simulink model "pathFollowing"  (R2023a)
settings: Solver=FixedStepDiscrete  StartTime=0.0  StopTime=Inf  FixedStep=0.1  RelTol=1e-3  EnableMultiTasking=on
StopFcn:
  | 
  |  % Do not delete, this is an auto-generated function to log ROS message.
  |  ros.slros.internal.ROSUtil.logROSMessageToBagFile(bdroot);
model workspace (MAT data in the model file):
  ROSLoggingInfo_.GenBagFile = 1
  ROSLoggingInfo_.BagFileName = 'pathFollowing'
  ROSLoggingInfo_.CompressionFormat = 'uncompressed'
  ROSLoggingInfo_.ChunkSize = 786432
  ROSLoggingInfo_.LogOption = 'Default'
  ROSLoggingInfo_.FilePrefix = ''
  ROSLoggingReload_{1,1} = 'pathFollowing/Altitude controller/Subscribe1'
  ROSLoggingReload_{2,1} = 'pathFollowing/Cameras/Subscribe2'
  ROSLoggingReload_{3,1} = 'pathFollowing/Cameras/Subscribe3'
  ROSLoggingReload_{4,1} = 'pathFollowing/Output/Blank Message'
  ROSLoggingReload_{5,1} = 'pathFollowing/Robot position/Subscribe1'
  ROSLoggingReload_{6,1} = 'pathFollowing/Altitude controller/Extract Position.Z/Msg'
  ROSLoggingReload_{7,1} = 'pathFollowing/Output/Bus
    | Assignment'
  ROSLoggingReload_{8,1} = 'pathFollowing/Robot position/Subsystem/In1'
  ROSLoggingReload_{1,2} = 0
  ROSLoggingReload_{2,2} = 0
  ROSLoggingReload_{3,2} = 0
  ROSLoggingReload_{4,2} = 0
  ROSLoggingReload_{5,2} = 1
  ROSLoggingReload_{6,2} = 0
  ROSLoggingReload_{7,2} = 0
  ROSLoggingReload_{8,2} = 0
  ROSLoggingReload_{1,3} = 'quadrotor_1_ground_truth_state_altitude_controller_subscribe1'
  ROSLoggingReload_{2,3} = 'quadrotor_1_front_image_raw_cameras_subscribe2'
  ROSLoggingReload_{3,3} = 'quadrotor_1_bottom_image_raw_cameras_subscribe3'
  ROSLoggingReload_{4,3} = 'output_blank_message'
  ROSLoggingReload_{5,3} = 'quadrotor_1_ground_truth_state_robot_position_subscribe1'
  ROSLoggingReload_{6,3} = []
  ROSLoggingReload_{7,3} = 'quadrotor_1/cmd_vel_output_bus_assignment'
  ROSLoggingReload_{8,3} = 'robot_position_subsystem_in1'
  ROSLoggingTable_ = {1, 'Robot position/Subscribe1:2', 'quadrotor_1_ground_truth_state_robot_position_subscribe1', 'nav_msgs/Odometry'}
  SL_ROS_VariableLengthArrays_MaxSizes.CommonInfo.ArrayTruncateAction = 'EmitWarning'
  SL_ROS_VariableLengthArrays_MaxSizes.MsgTypeMap = containers.Map
  SL_ROS_VariableLengthArrays_MaxSizes.MsgTypeMap.serialization.keys = {'sensor_msgs/Image', 'sensor_msgs/LaserScan'}
  SL_ROS_VariableLengthArrays_MaxSizes.MsgTypeMap.serialization.values{1}(1).PropertyName = 'Data'
  SL_ROS_VariableLengthArrays_MaxSizes.MsgTypeMap.serialization.values{1}(1).DataType = 'uint8'
  SL_ROS_VariableLengthArrays_MaxSizes.MsgTypeMap.serialization.values{1}(1).MaxLength = 691200
  SL_ROS_VariableLengthArrays_MaxSizes.MsgTypeMap.serialization.values{1}(2).PropertyName = 'Encoding'
  SL_ROS_VariableLengthArrays_MaxSizes.MsgTypeMap.serialization.values{1}(2).DataType = 'uint8'
  SL_ROS_VariableLengthArrays_MaxSizes.MsgTypeMap.serialization.values{1}(2).MaxLength = 128
  SL_ROS_VariableLengthArrays_MaxSizes.MsgTypeMap.serialization.values{2}(1).PropertyName = 'Intensities'
  SL_ROS_VariableLengthArrays_MaxSizes.MsgTypeMap.serialization.values{2}(1).DataType = 'single'
  SL_ROS_VariableLengthArrays_MaxSizes.MsgTypeMap.serialization.values{2}(1).MaxLength = 1081
  SL_ROS_VariableLengthArrays_MaxSizes.MsgTypeMap.serialization.values{2}(2).PropertyName = 'Ranges'
  SL_ROS_VariableLengthArrays_MaxSizes.MsgTypeMap.serialization.values{2}(2).DataType = 'single'
  SL_ROS_VariableLengthArrays_MaxSizes.MsgTypeMap.serialization.values{2}(2).MaxLength = 1081
  SL_ROS_VariableLengthArrays_MaxSizes.MsgTypeMap.serialization.uniformity = 0
  SL_ROS_VariableLengthArrays_MaxSizes.MsgTypeMap.serialization.keyType = 'char'
  SL_ROS_VariableLengthArrays_MaxSizes.MsgTypeMap.serialization.valueType = 'any'
undefined symbols (not defined in the file): Angular, gray, Linear
libraries: robotlib x8, slpidlib x1, robotalgslib x1, aerolibanimutils x1
settings Model: Creator=The MathWorks, Inc.  LastModifiedBy=root
settings SolverCC: AlgebraicLoopSolver=TrustRegion
settings DataIOCC: LimitDataPoints=on  SaveFormat=Array  ReturnWorkspaceOutputs=off
settings OptimizationCC: LifeSpan=Inf  MaxStackSize=64
settings DebuggingCC: SolverPrmCheckMsg=warning  UnconnectedInputMsg=warning  UnconnectedOutputMsg=warning  UnconnectedLineMsg=warning  SFUnexpectedBacktrackingDiag=warning  SFNoUnconditionalDefaultTransitionDiag=warning  SFExecutionAtInitializationDiag=none  ArithmeticOperatorsInVariantConditions=warning
settings HardwareCC: ProdBitPerPointer=32  ProdBitPerSizeT=32  ProdBitPerPtrDiffT=32  ProdLargestAtomicFloat=None  ProdIntDivRoundTo=Undefined  ProdEndianess=Unspecified  ProdWordSize=32  ProdHWDeviceType=Generic->Unspecified (assume 32-bit Generic)  UseEmbeddedCoderFeatures=off
settings ModelReferenceCC: EnableRefExpFcnMdlSchedulingChecks=on  PropagateSignalLabelsOutOfModel=off
settings SFSimCC: SimUseLocalCustomCode=off  CustomCodeUndefinedFunction=UseInterfaceOnly  SimTargetLang=C++
settings RTWCC: Description=Embedded Coder  SystemTargetFile=ert.tlc  HardwareBoard=Robot Operating System (ROS)  TLCOptions=-aInlineSetEventsForThisBaseRateFcn=TLC_FALSE -aSuppressMultiTaskScheduler=TLC_FALSE -aRateBasedStepFcn=0  TemplateMakefile=ert_default_tmf  RTWUseLocalCustomCode=off  Toolchain=Catkin  TargetLang=C++
settings CodeAppCC: StateflowObjectComments=on
settings ERTTargetCC: MultiwordLength=2048  ERTCustomFileBanners=off  SupportContinuousTime=on  SupportNonInlinedSFcns=on  RemoveResetFunc=off  SupportVariableSizeSignals=on  ModelStepFunctionPrototypeControlCompliant=off  ConvertIfToSwitch=off  SuppressUnreachableDefaultCases=off
settings ConfigComp: CovMetricSettings=dw  CovSaveCumulativeToWorkspaceVar=on  CovSaveSingleToWorkspaceVar=on  CovExternalEMLEnable=off  CovSFcnEnable=off

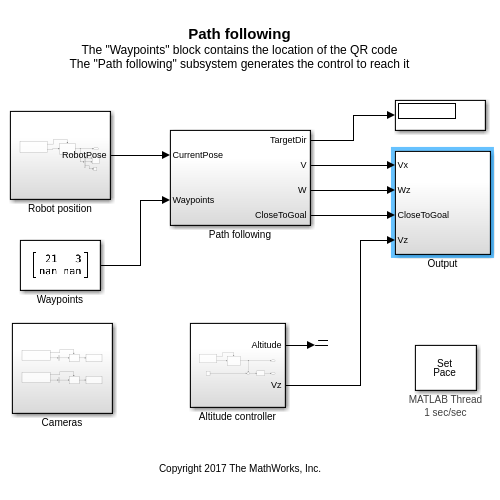
[thumbnail: Simulink's stored preview of the top-level diagram]
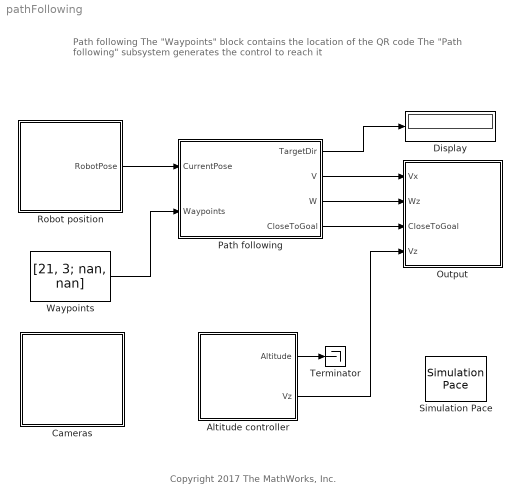
== system pathFollowing ==
  note: Path following
      | The "Waypoints" block contains the location of the QR code
      | The "Path following" subsystem generates the control to reach it
  note: Copyright 2017 The MathWorks, Inc.
  Altitude controller : Subsystem
  Cameras : Subsystem
  Display : Display
  Output : Subsystem
  Path following : Subsystem
  Robot position : Subsystem
  Simulation Pace : aerolibanimutils/Simulation Pace  SimulationPace=1  SleepMode=MATLAB Thread  OutputPaceError=off  SampleTime=-1
  Terminator : Terminator
  Waypoints : Constant  Value=[21, 3; nan, nan]  OutDataTypeStr=double
  wires:
  Waypoints/1 -> Path following/2(Waypoints)
  Path following/2(V) -> Output/1(Vx)
  Path following/4(CloseToGoal) -> Output/3(CloseToGoal)
  Path following/3(W) -> Output/2(Wz)
  Path following/1(TargetDir) -> Display/1
  Robot position/1(RobotPose) -> Path following/1(CurrentPose)
  Altitude controller/2(Vz) -> Output/4(Vz)
  Altitude controller/1(Altitude) -> Terminator/1

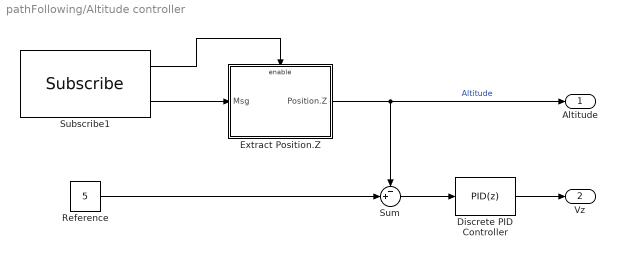
== system pathFollowing/Altitude controller ==
  Discrete PID Controller : slpidlib/PID Controller  Controller=PID  Form=Parallel  TimeDomain=Discrete-time  UseExternalTs=off  SampleTime=-1  IntegratorMethod=Forward Euler  FilterMethod=Forward Euler  ControllerParametersSource=internal  P=1  I=0  UseKiTs=off  D=0  N=100  UseFilter=on  TunerSelectOption=Transfer Function Based (PID Tuner App)  InitialConditionSource=internal  InitialConditionForIntegrator=0  InitialConditionForFilter=0  DifferentiatorICPrevScaledInput=0  ExternalReset=none  TrackingMode=off  Kt=1  LimitOutput=on  SatLimitsSource=internal  UpperSaturationLimit=1  LowerSaturationLimit=-1  LinearizeAsGain=off  AntiWindupMode=none  Kb=1  LimitIntegrator=off  UpperIntegratorSaturationLimit=inf  LowerIntegratorSaturationLimit=-inf  POutMin=[]  POutMax=[]  IOutMin=[]  IOutMax=[]  DOutMin=[]  DOutMax=[]  NOutMin=[]  NOutMax=[]  SumOutMin=[]  SumOutMax=[]  SaturationOutMin=[]  SaturationOutMax=[]  PParamMin=[]  PParamMax=[]  IParamMin=[]  IParamMax=[]  DParamMin=[]  DParamMax=[]  NParamMin=[]  NParamMax=[]  KbParamMin=[]  KbParamMax=[]  KtParamMin=[]  KtParamMax=[]  KbOutMin=[]  KbOutMax=[]  KtOutMin=[]  KtOutMax=[]  IntegratorOutMin=[]  IntegratorOutMax=[]  FilterOutMin=[]  FilterOutMax=[]  SumI1OutMin=[]  SumI1OutMax=[]  SumI2OutMin=[]  SumI2OutMax=[]  SumI3OutMin=[]  SumI3OutMax=[]  SumI4OutMin=[]  SumI4OutMax=[]  SumDOutMin=[]  SumDOutMax=[]  DifferentiatorOutMin=[]  DifferentiatorOutMax=[]  FilterDiffOutCoefMin=[]  FilterDiffOutCoefMax=[]  ReciprocalOutMin=[]  ReciprocalOutMax=[]  SumDenOutMin=[]  SumDenOutMax=[]  SumNumOutMin=[]  SumNumOutMax=[]  DivideOutMin=[]  DivideOutMax=[]  UdiffTsProdOutMin=[]  UdiffTsProdOutMax=[]  NTsProdOutMin=[]  NTsProdOutMax=[]  UintegralTsProdOutMin=[]  UintegralTsProdOutMax=[]  UngainTsProdOutMin=[]  UngainTsProdOutMax=[]  ClampingZeroOutDataTypeStr=Inherit: Inherit via back propagation  ClampingZeroOutMin=[]  ClampingZeroOutMax=[]  FilterDenConstantOutDataTypeStr=Inherit: Inherit via back propagation  FilterDenConstantOutMin=[]  FilterDenConstantOutMax=[]  PCopyOutDataTypeStr=Inherit: Inherit via back propagation  PCopyOutMin=[]  PCopyOutMax=[]  NCopyOutDataTypeStr=Inherit: Inherit via back propagation  NCopyOutMin=[]  NCopyOutMax=[]  IntegratorContinuousStateAttributes=''  IntegratorStateMustResolveToSignalObject=off  IntegratorRTWStateStorageClass=Auto  FilterContinuousStateAttributes=''  FilterStateMustResolveToSignalObject=off  FilterRTWStateStorageClass=Auto  ParallelPVariant=InternalParameters  IdealPVariant=Disabled  IVariant=InternalParameters  DVariant=InternalParameters  IntegratorVariant=Discrete  SatVariant=Enabled  AWVariant=Passthrough  PCopyVariant=Disabled  TRVariant=Disabled  FdbkBlocksVariant=Forward  IdealPFdbkVariant=Disabled  SatFdbkVariant=Disabled  DerivativeFilterVariant=ForwardEulerFilter  NVariant=InternalParameters  NCopyVariant=Disabled  FilterICVariant=InternalICsFilter  IntegratorICVariant=InternalICs  ExternalResetVariant=Disabled  TRSumVariant=Passthrough  SumFdbkVariant=Disabled  SumVariant=Sum_PID  TsampFilterVariant=InternalTs  TsampNgainVariant=Passthrough  TsampIntegralVariant=Disabled_SignalSpec  ExternalSaturationOutDataTypeStr=Inherit: Same as second input
  Extract Position.Z : Subsystem
  Reference : Constant  Value=5
  Subscribe1 : robotlib/Subscribe  topicSource=Select from ROS network  topic=/quadrotor_1/ground_truth/state  messageType=nav_msgs/Odometry  SampleTime=-1  legacyBusStruct=off  messageQueueLength=51
  Sum : Sum  Inputs=-+|
  Altitude : Outport
  Vz : Outport  Port=2
  wires:
  Subscribe1/1 -> Extract Position.Z/Enable
  Subscribe1/2 -> Extract Position.Z/1(Msg)
  Sum/1 -> Discrete PID Controller/1
  Reference/1 -> Sum/2
  Extract Position.Z/1(Position.Z) -> Altitude/1, Sum/1  "Altitude"
  Discrete PID Controller/1 -> Vz/1

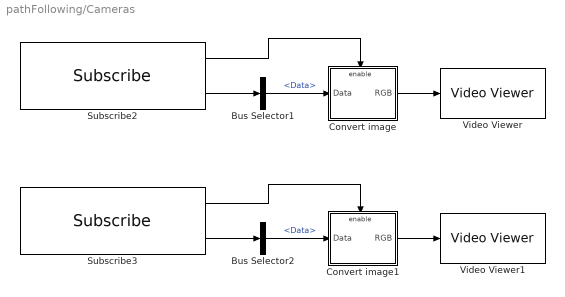
== system pathFollowing/Cameras ==
  Bus Selector1 : BusSelector  DialogController=Simulink.DDGSource_BusSelector  OutputSignals=Data
  Bus Selector2 : BusSelector  DialogController=Simulink.DDGSource_BusSelector  OutputSignals=Data
  Convert image : Subsystem
  Convert image1 : Subsystem
  Subscribe2 : robotlib/Subscribe  topicSource=Select from ROS network  topic=/quadrotor_1/front/image_raw  messageType=sensor_msgs/Image  SampleTime=-1  legacyBusStruct=off  messageQueueLength=51
  Subscribe3 : robotlib/Subscribe  topicSource=Select from ROS network  topic=/quadrotor_1/bottom/image_raw  messageType=sensor_msgs/Image  SampleTime=-1  legacyBusStruct=off  messageQueueLength=51
  Video Viewer : VideoViewer  colormapValue=gray(256)  FigPos=[252 563 599 376]
  Video Viewer1 : VideoViewer  colormapValue=gray(256)  FigPos=[964 607 629 376]
  wires:
  Subscribe2/1 -> Convert image/Enable
  Convert image1/1(RGB) -> Video Viewer1/1
  Subscribe3/2 -> Bus Selector2/1
  Subscribe2/2 -> Bus Selector1/1
  Bus Selector1/1 -> Convert image/1(Data)  "<Data>"
  Bus Selector2/1 -> Convert image1/1(Data)  "<Data>"
  Subscribe3/1 -> Convert image1/Enable
  Convert image/1(RGB) -> Video Viewer/1

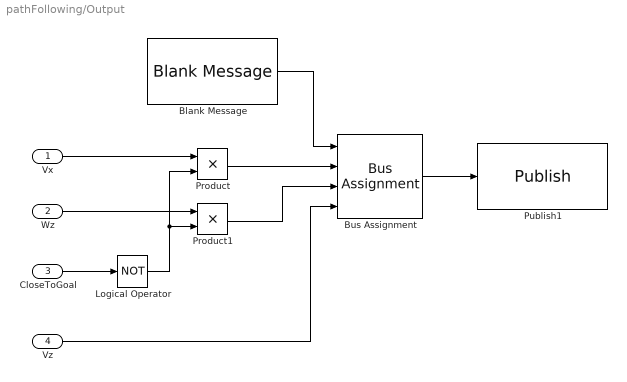
== system pathFollowing/Output ==
  Vx : Inport
  Wz : Inport  Port=2
  CloseToGoal : Inport  Port=3
  Vz : Inport  Port=4
  Blank Message : robotlib/Blank Message  messageClass=Message  entityType=geometry_msgs/Twist  messageType=geometry_msgs/Twist  SampleTime=0  legacyBusStruct=off
  Bus Assignment : BusAssignment  DialogController=Simulink.DDGSource_BusAssignment  AssignedSignals=Linear.X,Angular.Z,Linear.Z
  Logical Operator : Logic  Operator=NOT  AllPortsSameDT=off  OutDataTypeStr=boolean
  Product : Product
  Product1 : Product
  Publish1 : robotlib/Publish  topicSource=Select from ROS network  topic=/quadrotor_1/cmd_vel  messageType=geometry_msgs/Twist  legacyBusStruct=off  messageQueueLength=105
  wires:
  Bus Assignment/1 -> Publish1/1
  Blank Message/1 -> Bus Assignment/1
  Logical Operator/1 -> Product1/2, Product/2
  Product1/1 -> Bus Assignment/3
  CloseToGoal/1 -> Logical Operator/1
  Product/1 -> Bus Assignment/2
  Vx/1 -> Product/1
  Wz/1 -> Product1/1
  Vz/1 -> Bus Assignment/4

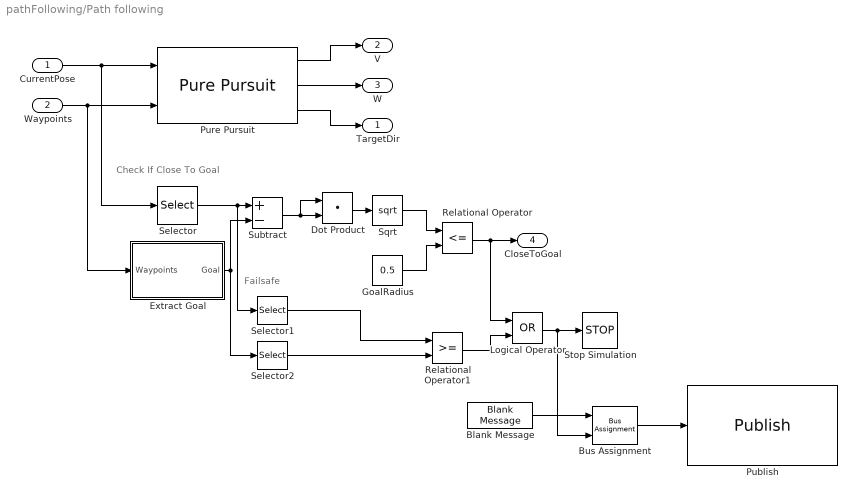
== system pathFollowing/Path following ==
  note: Check If Close To Goal
  note: Failsafe
  CurrentPose : Inport
  Waypoints : Inport  Port=2
  " Extract Goal" : MATLAB Function  TreatAsAtomicUnit=on
  Blank Message : robotlib/Blank Message  messageClass=Message  entityType=std_msgs/Bool  messageType=std_msgs/Bool  SampleTime=inf  legacyBusStruct=off
  Bus Assignment : BusAssignment  AssignedSignals=Data
  Dot Product : DotProduct  OutDataTypeStr=Inherit: Inherit via internal rule
  GoalRadius : Constant  Value=0.5
  Logical Operator : Logic  Operator=OR  AllPortsSameDT=off  OutDataTypeStr=boolean
  Publish : robotlib/Publish  topicSource=Specify your own  topic=/pause_gazebo_topic  messageType=std_msgs/Bool  legacyBusStruct=off  messageQueueLength=1
  Pure Pursuit : robotalgslib/Pure Pursuit  DesiredLinearVelocity=0.3  MaxAngularVelocity=1.0  LookaheadDistance=2.0  TargetDirPort=on  SimulateUsing=Code generation
  Relational Operator : RelationalOperator  Operator=<=  OutDataTypeStr=boolean  RndMeth=Simplest  InputSameDT=off
  Relational Operator1 : RelationalOperator  OutDataTypeStr=boolean  RndMeth=Simplest  InputSameDT=off
  Selector : Selector  InputPortWidth=3  IndexOptions=Index vector (dialog)  Indices=[1 2]  OutputSizes=1
  Selector1 : Selector  InputPortWidth=2  IndexOptions=Index vector (dialog)  Indices=[1]  OutputSizes=1
  Selector2 : Selector  InputPortWidth=2  IndexOptions=Index vector (dialog)  Indices=[1]  OutputSizes=1
  Sqrt : Sqrt
  Stop Simulation : Stop
  Subtract : Sum  Inputs=+-
  TargetDir : Outport
  V : Outport  Port=2
  W : Outport  Port=3
  CloseToGoal : Outport  Port=4
  wires:
  Pure Pursuit/3 -> TargetDir/1
  Pure Pursuit/2 -> W/1
  Pure Pursuit/1 -> V/1
  " Extract Goal"/1(Goal) -> Subtract/2, Selector2/1
  Waypoints/1 -> " Extract Goal"/1(Waypoints), Pure Pursuit/2
  CurrentPose/1 -> Selector/1, Pure Pursuit/1
  GoalRadius/1 -> Relational Operator/2
  Selector/1 -> Selector1/1, Subtract/1
  Dot Product/1 -> Sqrt/1
  Sqrt/1 -> Relational Operator/1
  Subtract/1 -> Dot Product/1, Dot Product/2
  Relational Operator/1 -> Logical Operator/1, CloseToGoal/1
  Logical Operator/1 -> Bus Assignment/2, Stop Simulation/1
  Selector1/1 -> Relational Operator1/1
  Selector2/1 -> Relational Operator1/2
  Relational Operator1/1 -> Logical Operator/2
  Blank Message/1 -> Bus Assignment/1
  Bus Assignment/1 -> Publish/1

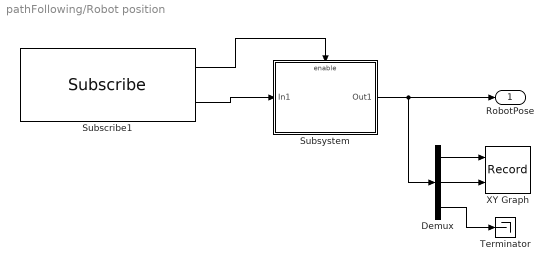
== system pathFollowing/Robot position ==
  Demux : Demux  Outputs=3
  Subscribe1 : robotlib/Subscribe  topicSource=Select from ROS network  topic=/quadrotor_1/ground_truth/state  messageType=nav_msgs/Odometry  SampleTime=-1  legacyBusStruct=off  messageQueueLength=51
  Subsystem : Subsystem
  Terminator : Terminator
  XY Graph : Record  FileSettingsInternal="{\"entries\":[{\"content\":{\"excelSettings\":{\"content\":{},\"type\":\"Streamout.ExcelSettings\"}},\"type\":\"Streamout.FileSettingStorage\",\"uuid\":\"\"}],\"packageUris\":[\"http:\\/\\/schema.mathworks.com\\/mf0\\/streamout_blocks\\/R2020a\"],\"version\":\"1.0\"}"  Layout=[1 1]  SignalsInternal="{\"entries\":[{\"content\":{\"signals\":[{\"content\":{\"blockPath\":[],\"dimensions\":[1],\"domain\":\"\",\"lineColor\":\"#a2142f\",\"plots\":[1],\"port\":1,\"signalID\":34,\"signalName\":\"Demux:1\"},\"type\":\"RecordBlkView.Signal\",\"uuid\":\"\"},{\"content\":{\"blockPath\":[],\"dimensions\":[1],\"domain\":\"\",\"lineColor\":\"#139fff\",\"plots\":[1],\"port\":2,\"signalID\":37,\"signalName\":\"Demux:2\"},\"type\":\"RecordBlkView.Signal\",\"uuid\":\"\"}]},\"type\":\"RecordBlkView.InputSignals\",\"uuid\":\"\"}],\"packageUris\":[\"http:\\/\\/schema.mathworks.com\\/mf0\\/streamout_blocks\\/R2020a\"],\"version\":\"1.0\"}"  VisualizationBindings="{\"xyplotplugin\":{\"info\":[{\"series\":[{\"bindingParametersList\":[{\"parameter\":\"X-Axis\",\"signalID\":34,\"signalName\":\"Demux:1\"},{\"parameter\":\"Y-Axis\",\"signalID\":37,\"signalName\":\"Demux:2\"}],\"seriesID\":62390}],\"subplotID\":1}]}}"  CompatibilityTag=XY  st=-1
  RobotPose : Outport
  wires:
  Subscribe1/1 -> Subsystem/Enable
  Subscribe1/2 -> Subsystem/1(In1)
  Subsystem/1(Out1) -> Demux/1, RobotPose/1
  Demux/2 -> XY Graph/2
  Demux/1 -> XY Graph/1
  Demux/3 -> Terminator/1

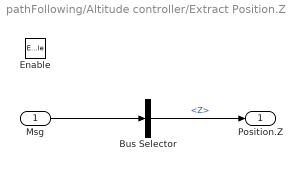
== system pathFollowing/Altitude controller/Extract Position.Z ==
  Msg : Inport
  Enable : EnablePort
  Bus Selector : BusSelector  OutputSignals=Pose.Pose.Position.Z
  Position.Z : Outport
  wires:
  Msg/1 -> Bus Selector/1
  Bus Selector/1 -> Position.Z/1  "<Z>"

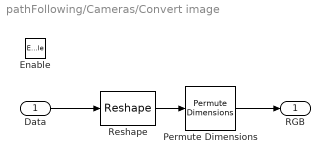
== system pathFollowing/Cameras/Convert image ==
  Data : Inport
  Enable : EnablePort
  Permute Dimensions : PermuteDimensions  Order=[3 2 1]
  Reshape : Reshape  OutputDimensionality=Customize  OutputDimensions=[3 640 360]
  RGB : Outport
  wires:
  Permute Dimensions/1 -> RGB/1
  Reshape/1 -> Permute Dimensions/1
  Data/1 -> Reshape/1

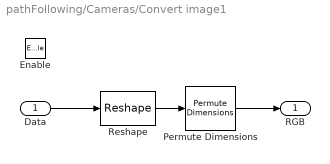
== system pathFollowing/Cameras/Convert image1 ==
  Data : Inport
  Enable : EnablePort
  Permute Dimensions : PermuteDimensions  Order=[3 2 1]
  Reshape : Reshape  OutputDimensionality=Customize  OutputDimensions=[3 640 360]
  RGB : Outport
  wires:
  Permute Dimensions/1 -> RGB/1
  Reshape/1 -> Permute Dimensions/1
  Data/1 -> Reshape/1

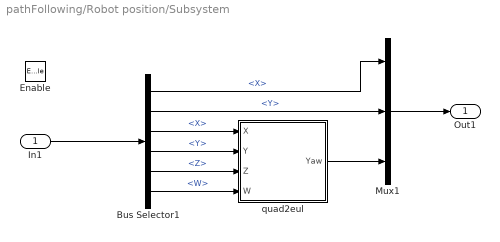
== system pathFollowing/Robot position/Subsystem ==
  In1 : Inport
  Enable : EnablePort
  Bus Selector1 : BusSelector  OutputSignals=Pose.Pose.Position.X,Pose.Pose.Position.Y,Pose.Pose.Orientation.X,Pose.Pose.Orientation.Y,Pose.Pose.Orientation.Z,Pose.Pose.Orientation.W
  Mux1 : Mux  Inputs=3
  quad2eul : MATLAB Function  TreatAsAtomicUnit=on
  Out1 : Outport
  wires:
  Bus Selector1/5 -> quad2eul/3(Z)  "<Z>"
  Bus Selector1/4 -> quad2eul/2(Y)  "<Y>"
  Bus Selector1/3 -> quad2eul/1(X)  "<X>"
  Bus Selector1/2 -> Mux1/2  "<Y>"
  quad2eul/1(Yaw) -> Mux1/3
  Mux1/1 -> Out1/1
  Bus Selector1/6 -> quad2eul/4(W)  "<W>"
  Bus Selector1/1 -> Mux1/1  "<X>"
  In1/1 -> Bus Selector1/1

== matlab function pathFollowing/Robot position/Subsystem/quad2eul ==
  data: X input; Yaw output; Y input; Z input; W input
function Yaw = quat2eulBlk(X, Y, Z, W)
%#codegen

eularAngles = quat2eul([W, X, Y, Z]);
Yaw = eularAngles(1);

== matlab function pathFollowing/Path following/ Extract Goal ==
  data: Waypoints input; Goal output
function Goal = extractGoal(Waypoints)
%#codegen
b = isnan(Waypoints);
[rows,~] = find(b);
ridx = setdiff(1:size(Waypoints,1), sort(rows));
Goal = [Waypoints(ridx(end), 1) Waypoints(ridx(end), 2)];
